simulink model "Lab4_jinjin"  (R2022a)
settings: Solver=VariableStepAuto  StartTime=0.0  StopTime=1200  RelTol=1e-3
libraries: sharedutil x2
settings Model: Creator=Administrator  LastModifiedBy=이진진
settings DebuggingCC: UnconnectedInputMsg=warning  UnconnectedOutputMsg=warning  UnconnectedLineMsg=warning
settings RTWCC: DLArmComputeVersion=19.05

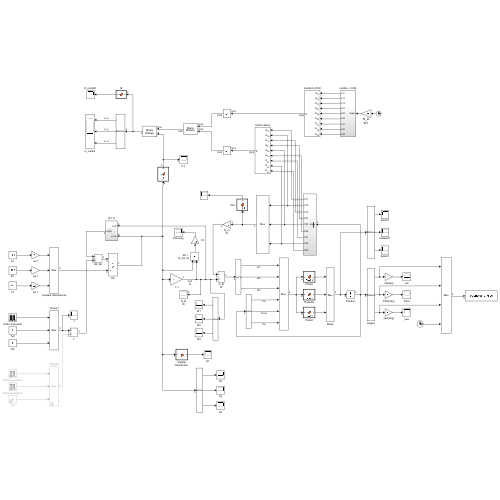
[thumbnail: Simulink's stored preview of the top-level diagram]
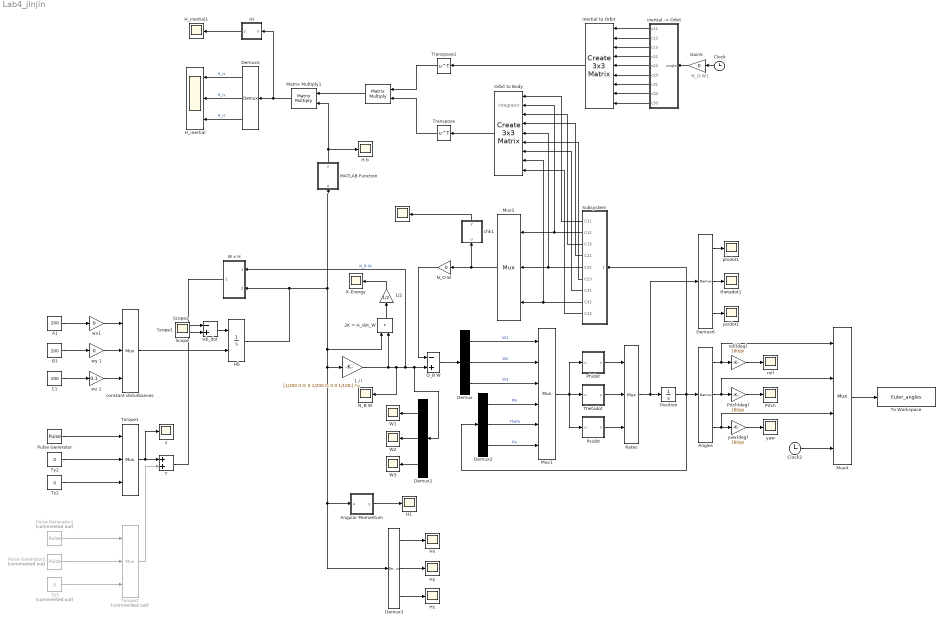
== system Lab4_jinjin ==
  note: N_O
      | W1
  note: integrator
  " " : Scope
  "  " : Product  Multiplication=Matrix(*)
  1 : Scope
  1 / I : Gain  Gain=[1/200 0 0; 0 1/200 0; 0 0 1/100;]  Multiplication=Matrix(K*u)
  1/2 : Gain  Gain=1/2
  2K = H_dot_W : DotProduct  OutDataTypeStr=Inherit: Inherit via internal rule
  A1 : Constant  Value=200
  Angles : Demux  Outputs=3
      settings: DisplayOption=none
  Angular Momentum : MATLAB Function  TreatAsAtomicUnit=on
  B1 : Constant  Value=200
  C1 : Constant  Value=100
  Clock : Clock
  Clock2 : Clock
  Demux{,1..3,5..6} (6 alike) : Demux  Outputs=3
      settings: DisplayOption=none
  Gain5 : Gain  Gain=0
  H b : Scope
  H1 : Scope
  HI : MATLAB Function  TreatAsAtomicUnit=on
  H_inertial : Scope  NumInputPorts=3
  H_inertial1 : Scope
  Hb : Integrator  InitialConditionSource=external  InitialCondition=[0.2;0.3;0.4]
  Hb_dot : Sum  Inputs=-+
  Hx : Scope
  Hy : Scope
  Hz : Scope
  Inertial to Orbit : sharedutil/Create 3x3 Matrix  aMode=aMode
      settings: SourceProductBaseCode=AE,PW,DR,MT,VE
  K-Energy : Scope
  MATLAB Function : MATLAB Function  TreatAsAtomicUnit=on
  Matrix Multiply1 : Product  Multiplication=Matrix(*)
  Mux1 : Mux  Inputs=6
  Mux2 : Mux  Inputs=3
  Mux4 : Mux
  N_B W : Scope
  N_O W : Gain  Gain=0
  O_B W : Sum  Inputs=-+
  Orbit to Body : sharedutil/Create 3x3 Matrix  aMode=aMode
      settings: SourceProductBaseCode=AE,PW,DR,MT,VE
  Phidot : MATLAB Function  TreatAsAtomicUnit=on
  Pitch : Scope
  Pitch(deg) : Gain  Gain=180/pi
  Position : Integrator  InitialCondition=[0 0 0]
  Psidot : MATLAB Function  TreatAsAtomicUnit=on
  Pulse Generator : DiscretePulseGenerator  PulseType=Time based  Amplitude=300  Period=10000  PulseWidth=0.0001  PhaseDelay=100
  Pulse Generator1 : DiscretePulseGenerator  Commented=on  PulseType=Time based  Amplitude=287.35  Period=10000  PulseWidth=0.0001  PhaseDelay=157.6
  Pulse Generator2 : DiscretePulseGenerator  Commented=on  PulseType=Time based  Amplitude=86.21  Period=10000  PulseWidth=0.0001  PhaseDelay=157.6
  Rates : Mux  Inputs=3
  Subsystem : Subsystem
  T : Sum
  Thetadot : MATLAB Function  TreatAsAtomicUnit=on
  To Workspace : ToWorkspace  VariableName=Euler_angles  SampleTime=-1
  Torque1 : Mux  Inputs=3
  Torque2 : Mux  Commented=on  Inputs=3
  Transpose : Math  Operator=transpose
  Transpose1 : Math  Operator=transpose
  Ty2 : Constant  Value=0
  Tz2 : Constant  Value=0
  Tz3 : Constant  Commented=on  Value=0
  W x H : Subsystem
  W1 : Scope
  W2 : Scope
  W3 : Scope
  chk1 : MATLAB Function  TreatAsAtomicUnit=on
  constant disturbances : Mux  Inputs=3
  "inertial -> Orbit" : Subsystem
  phidot1 : Scope
  psidot1 : Scope
  roll : Scope
  roll(deg) : Gain  Gain=180/pi
  thetadot1 : Scope
  wx1 : Gain  Gain=0
  wy 1 : Gain  Gain=0
  wz 1 : Gain  Gain=0.1
  yaw : Scope
  yaw(deg) : Gain  Gain=180/pi
  Scope : Scope
  Scope1 : Scope
  Scope2 : Scope
  wires:
  Hb_dot/1 -> Hb/1
  W x H/1(WxH) -> Hb_dot/1
  Position/1 -> Demux2/1, Subsystem/1(angle), Angles/1
  Rates/1 -> Position/1, Demux6/1
  Thetadot/1(y) -> Rates/2
  Demux2/1 -> Mux1/4  "Phi"
  Phidot/1(y) -> Rates/1
  Demux2/3 -> Mux1/6  "Psi"
  Demux1/2 -> W2/1
  Demux/3 -> Mux1/3  "W3"
  O_B W/1 -> Demux/1
  Subsystem/2(C12) -> Mux2/1, Orbit to Body/2
  roll(deg)/1 -> roll/1
  Angles/2 -> Mux4/2, Pitch(deg)/1
  yaw(deg)/1 -> yaw/1
  Angles/1 -> Mux4/1, roll(deg)/1
  Demux/2 -> Mux1/2  "W2"
  "  "/1 -> Matrix Multiply1/1
  Subsystem/1(C11) -> Orbit to Body/1
  Transpose/1 -> "  "/2
  Subsystem/4(C21) -> Orbit to Body/4
  1 / I/1 -> N_B W/1, W x H/1(in W), Demux1/1, O_B W/2, 2K = H_dot_W/2  "N_B W"
  Transpose1/1 -> "  "/1
  Orbit to Body/1 -> Transpose/1
  Inertial to Orbit/1 -> Transpose1/1
  Demux1/3 -> W3/1
  Subsystem/9(C33) -> Orbit to Body/9
  "inertial -> Orbit"/5(c22) -> Inertial to Orbit/5
  Angles/3 -> Mux4/3, yaw(deg)/1
  Clock/1 -> Gain5/1
  2K = H_dot_W/1 -> 1/2/1
  chk1/1(y) -> " "/1
  Demux3/3 -> Hz/1
  Gain5/1 -> "inertial -> Orbit"/1(angle)
  "inertial -> Orbit"/8(c32) -> Inertial to Orbit/8
  Demux3/2 -> Hy/1
  Psidot/1(y) -> Rates/3
  Mux4/1 -> To Workspace/1
  Demux6/1 -> phidot1/1
  Demux6/2 -> thetadot1/1
  Pitch(deg)/1 -> Pitch/1
  "inertial -> Orbit"/7(c31) -> Inertial to Orbit/7
  "inertial -> Orbit"/3(c13) -> Inertial to Orbit/3
  Clock2/1 -> Mux4/4
  Subsystem/6(C23) -> Orbit to Body/6
  Mux2/1 -> chk1/1(u), N_O W/1
  Demux3/1 -> Hx/1
  Subsystem/5(C22) -> Orbit to Body/5, Mux2/2
  N_O W/1 -> O_B W/1
  "inertial -> Orbit"/4(c21) -> Inertial to Orbit/4
  Demux/1 -> Mux1/1  "W1"
  Angular Momentum/1(y) -> H1/1
  Demux2/2 -> Mux1/5  "Theta"
  Subsystem/7(C31) -> Orbit to Body/7
  "inertial -> Orbit"/2(c12) -> Inertial to Orbit/2
  Hb/1 -> Angular Momentum/1(u), Demux3/1, 1 / I/1, 2K = H_dot_W/1, MATLAB Function/1(u), W x H/2(in Hb)
  Demux6/3 -> psidot1/1
  Demux1/1 -> W1/1
  "inertial -> Orbit"/9(c33) -> Inertial to Orbit/9
  "inertial -> Orbit"/1(c11) -> Inertial to Orbit/1
  "inertial -> Orbit"/6(c23) -> Inertial to Orbit/6
  MATLAB Function/1(y) -> H b/1, Matrix Multiply1/2
  Mux1/1 -> Thetadot/1(u), Psidot/1(u), Phidot/1(u)
  Subsystem/8(C32) -> Orbit to Body/8, Mux2/3
  Subsystem/3(C13) -> Orbit to Body/3
  1/2/1 -> K-Energy/1
  C1/1 -> wz 1/1
  B1/1 -> wy 1/1
  Pulse Generator2/1 -> Torque2/2
  Tz3/1 -> Torque2/3
  constant disturbances/1 -> Hb/2
  wy 1/1 -> constant disturbances/2
  Ty2/1 -> Torque1/2
  wz 1/1 -> constant disturbances/3
  Torque2/1 -> T/2
  Pulse Generator1/1 -> Torque2/1
  A1/1 -> wx1/1
  Torque1/1 -> 1/1, T/1
  Tz2/1 -> Torque1/3
  wx1/1 -> constant disturbances/1
  Pulse Generator/1 -> Torque1/1
  T/1 -> Hb_dot/2
  Demux5/2 -> H_inertial/2  "H_iy"
  HI/1(y) -> H_inertial1/1
  Demux5/1 -> H_inertial/1  "H_ix"
  Matrix Multiply1/1 -> HI/1(u), Demux5/1
  Demux5/3 -> H_inertial/3  "H_iz"

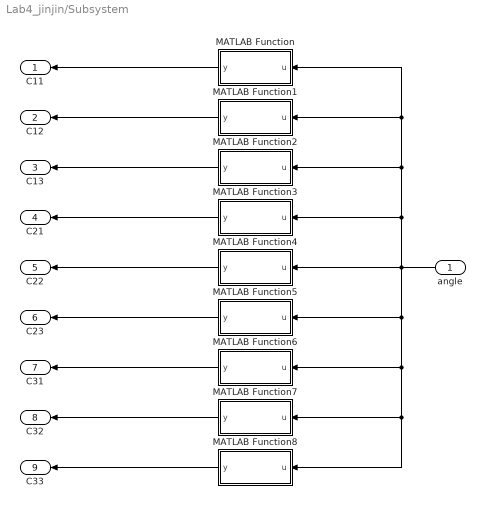
== system Lab4_jinjin/Subsystem ==
  angle : Inport
  MATLAB Function : MATLAB Function  TreatAsAtomicUnit=on
  MATLAB Function1 : MATLAB Function  TreatAsAtomicUnit=on
  MATLAB Function2 : MATLAB Function  TreatAsAtomicUnit=on
  MATLAB Function3 : MATLAB Function  TreatAsAtomicUnit=on
  MATLAB Function4 : MATLAB Function  TreatAsAtomicUnit=on
  MATLAB Function5 : MATLAB Function  TreatAsAtomicUnit=on
  MATLAB Function6 : MATLAB Function  TreatAsAtomicUnit=on
  MATLAB Function7 : MATLAB Function  TreatAsAtomicUnit=on
  MATLAB Function8 : MATLAB Function  TreatAsAtomicUnit=on
  C11 : Outport
  C12 : Outport  Port=2
  C13 : Outport  Port=3
  C21 : Outport  Port=4
  C22 : Outport  Port=5
  C23 : Outport  Port=6
  C31 : Outport  Port=7
  C32 : Outport  Port=8
  C33 : Outport  Port=9
  wires:
  MATLAB Function8/1(y) -> C33/1
  MATLAB Function7/1(y) -> C32/1
  MATLAB Function6/1(y) -> C31/1
  MATLAB Function5/1(y) -> C23/1
  MATLAB Function4/1(y) -> C22/1
  MATLAB Function3/1(y) -> C21/1
  MATLAB Function2/1(y) -> C13/1
  MATLAB Function1/1(y) -> C12/1
  MATLAB Function/1(y) -> C11/1
  angle/1 -> MATLAB Function/1(u), MATLAB Function1/1(u), MATLAB Function2/1(u), MATLAB Function3/1(u), MATLAB Function4/1(u), MATLAB Function5/1(u), MATLAB Function6/1(u), MATLAB Function7/1(u), MATLAB Function8/1(u)

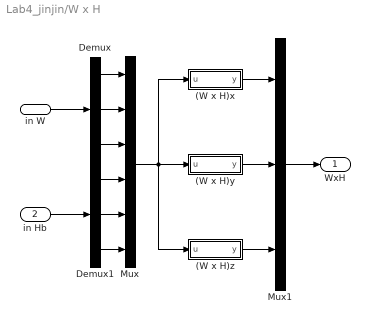
== system Lab4_jinjin/W x H ==
  in W : Inport
  in Hb : Inport  Port=2
  (W x H)x : MATLAB Function  TreatAsAtomicUnit=on
  (W x H)y : MATLAB Function  TreatAsAtomicUnit=on
  (W x H)z : MATLAB Function  TreatAsAtomicUnit=on
  Demux : Demux  Outputs=3
      settings: DisplayOption=none
  Demux1 : Demux  Outputs=3
      settings: DisplayOption=none
  Mux : Mux  Inputs=6
  Mux1 : Mux  Inputs=3
  WxH : Outport
  wires:
  in W/1 -> Demux/1
  in Hb/1 -> Demux1/1
  Demux1/1 -> Mux/4
  Demux1/2 -> Mux/5
  Demux1/3 -> Mux/6
  Demux/3 -> Mux/3
  Demux/2 -> Mux/2
  Demux/1 -> Mux/1
  Mux/1 -> (W x H)z/1(u), (W x H)x/1(u), (W x H)y/1(u)
  (W x H)x/1(y) -> Mux1/1
  (W x H)y/1(y) -> Mux1/2
  (W x H)z/1(y) -> Mux1/3
  Mux1/1 -> WxH/1

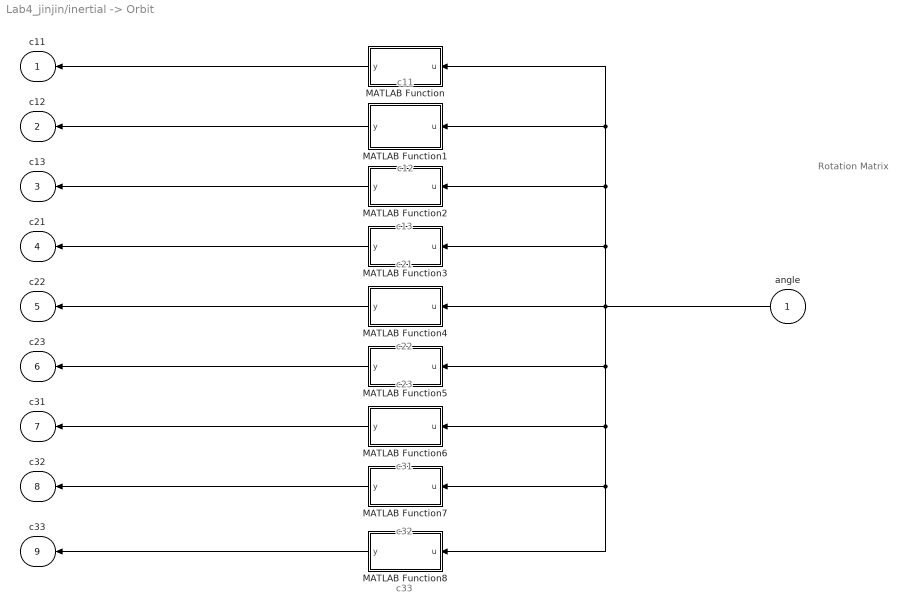
== system Lab4_jinjin/inertial -> Orbit ==
  note: c33
  note: c32
  note: c31
  note: c23
  note: c22
  note: c21
  note: c13
  note: c12
  note: Rotation Matrix
  note: c11
  angle : Inport
  MATLAB Function : MATLAB Function  TreatAsAtomicUnit=on
  MATLAB Function1 : MATLAB Function  TreatAsAtomicUnit=on
  MATLAB Function2 : MATLAB Function  TreatAsAtomicUnit=on
  MATLAB Function3 : MATLAB Function  TreatAsAtomicUnit=on
  MATLAB Function4 : MATLAB Function  TreatAsAtomicUnit=on
  MATLAB Function5 : MATLAB Function  TreatAsAtomicUnit=on
  MATLAB Function6 : MATLAB Function  TreatAsAtomicUnit=on
  MATLAB Function7 : MATLAB Function  TreatAsAtomicUnit=on
  MATLAB Function8 : MATLAB Function  TreatAsAtomicUnit=on
  c11 : Outport
  c12 : Outport  Port=2
  c13 : Outport  Port=3
  c21 : Outport  Port=4
  c22 : Outport  Port=5
  c23 : Outport  Port=6
  c31 : Outport  Port=7
  c32 : Outport  Port=8
  c33 : Outport  Port=9
  wires:
  MATLAB Function8/1(y) -> c33/1
  MATLAB Function7/1(y) -> c32/1
  MATLAB Function6/1(y) -> c31/1
  MATLAB Function5/1(y) -> c23/1
  MATLAB Function4/1(y) -> c22/1
  MATLAB Function3/1(y) -> c21/1
  MATLAB Function2/1(y) -> c13/1
  MATLAB Function1/1(y) -> c12/1
  MATLAB Function/1(y) -> c11/1
  angle/1 -> MATLAB Function2/1(u), MATLAB Function/1(u), MATLAB Function1/1(u), MATLAB Function3/1(u), MATLAB Function4/1(u), MATLAB Function5/1(u), MATLAB Function6/1(u), MATLAB Function7/1(u), MATLAB Function8/1(u)

== matlab function Lab4_jinjin/Thetadot ==
  data: u input; y output
function y = Thetadot(u)

y = cos(u(4))*u(2) - sin(u(4))*u(3);

end

== matlab function Lab4_jinjin/Angular Momentum ==
  data: u input; y output
function y = f(u)

y = sqrt(u(1)^2 + u(2)^2 + u(3)^2);

end

== matlab function Lab4_jinjin/chk1 ==
  data: u input; y output
function y = chk1(u)

y = sqrt(u(1)^2 + u(2)^2 + u(3)^2) - 1;

end

== matlab function Lab4_jinjin/inertial -> Orbit/MATLAB Function ==
  data: u input; y output
function y = fcn(u)

y = cos(u(1));

end

== matlab function Lab4_jinjin/inertial -> Orbit/MATLAB Function1 ==
  data: u input; y output
function y = fcn(u)

y = 0;

end

== matlab function Lab4_jinjin/W x H/(W x H)x ==
  data: u input; y output
function y = fcn(u)

y = u(2)*u(6) - u(3)*u(5);

== matlab function Lab4_jinjin/inertial -> Orbit/MATLAB Function2 ==
  data: u input; y output
function y = fcn(u)

y = -sin(u(1));

end

== matlab function Lab4_jinjin/inertial -> Orbit/MATLAB Function3 ==
  data: u input; y output
function y = fcn(u)

y = 0;

end

== matlab function Lab4_jinjin/inertial -> Orbit/MATLAB Function4 ==
  data: u input; y output
function y = fcn(u)

y = 1;

end

== matlab function Lab4_jinjin/inertial -> Orbit/MATLAB Function5 ==
  data: u input; y output
function y = fcn(u)

y = 0;

end

== matlab function Lab4_jinjin/inertial -> Orbit/MATLAB Function6 ==
  data: u input; y output
function y = fcn(u)

y = sin(u(1));

end

== matlab function Lab4_jinjin/inertial -> Orbit/MATLAB Function7 ==
  data: u input; y output
function y = fcn(u)

y = 0;
end

== matlab function Lab4_jinjin/inertial -> Orbit/MATLAB Function8 ==
  data: u input; y output
function y = fcn(u)

y = cos(u(1));

end

== matlab function Lab4_jinjin/MATLAB Function ==
  data: u input; y output
function y = f(u)

y = zeros(3,1);

y(1,1) = u(1);
y(2,1) = u(2);
y(3,1) = u(3);

== matlab function Lab4_jinjin/HI ==
  data: u input; y output
function y = fcn(u)

y = sqrt((u(1)^2+u(2)^2+u(3)^2));

== matlab function Lab4_jinjin/W x H/(W x H)z ==
  data: u input; y output
function y = fcn(u)

y = u(1)*u(5) - u(2)*u(4);

== matlab function Lab4_jinjin/Phidot ==
  data: u input; y output
function y = Phidot(u)

y = u(1) + sin(u(4))*tan(u(5))*u(2) + cos(u(4))*tan(u(5))*u(3);

end

== matlab function Lab4_jinjin/Psidot ==
  data: u input; y output
function y = Psidot(u)

y = (sin(u(4))/cos(u(5)))*u(2) + (cos(u(4))/cos(u(5))*u(3));

end

== matlab function Lab4_jinjin/Subsystem/MATLAB Function ==
  data: u input; y output
function y = C11(u)

y = cos(u(3))*cos(u(2));

end

== matlab function Lab4_jinjin/Subsystem/MATLAB Function1 ==
  data: u input; y output
function y = C12(u)

y = sin(u(3))*cos(u(2));

end

== matlab function Lab4_jinjin/Subsystem/MATLAB Function2 ==
  data: u input; y output
function y = C13(u)

y = -sin(u(2));

end

== matlab function Lab4_jinjin/Subsystem/MATLAB Function3 ==
  data: u input; y output
function y = C21(u)

y = -sin(u(3))*cos(u(1)) + cos(u(3))*sin(u(2))*sin(u(1));

end

== matlab function Lab4_jinjin/W x H/(W x H)y ==
  data: u input; y output
function y = fcn(u)

y = u(3)*u(4) - u(1)*u(6);

== matlab function Lab4_jinjin/Subsystem/MATLAB Function4 ==
  data: u input; y output
function y = C22(u)

y = cos(u(3))*cos(u(1)) + sin(u(3))*sin(u(2))*sin(u(1));

end

== matlab function Lab4_jinjin/Subsystem/MATLAB Function5 ==
  data: u input; y output
function y = C23(u)

y = cos(u(2))*sin(u(1));

end

== matlab function Lab4_jinjin/Subsystem/MATLAB Function6 ==
  data: u input; y output
function y = C31(u)

y = sin(u(3))*sin(u(1)) + cos(u(3))*sin(u(2))*cos(u(1));

end

== matlab function Lab4_jinjin/Subsystem/MATLAB Function7 ==
  data: u input; y output
function y = C32(u)

y = -cos(u(3))*sin(u(1)) + sin(u(3))*sin(u(2))*cos(u(1));

end

== matlab function Lab4_jinjin/Subsystem/MATLAB Function8 ==
  data: u input; y output
function y = C33(u)

y = cos(u(2))*cos(u(1));

end
